simulink model "Motor_Postion_Ctrl"  (R2020a)
settings: Solver=VariableStepAuto  StartTime=0.0  StopTime=10.0  RelTol=1e-3
undefined symbols (not defined in the file): b, J, K, L, R
settings Model: DataDictionary=Motor_data.sldd  Creator=NIKITA  LastModifiedBy=NIKITA

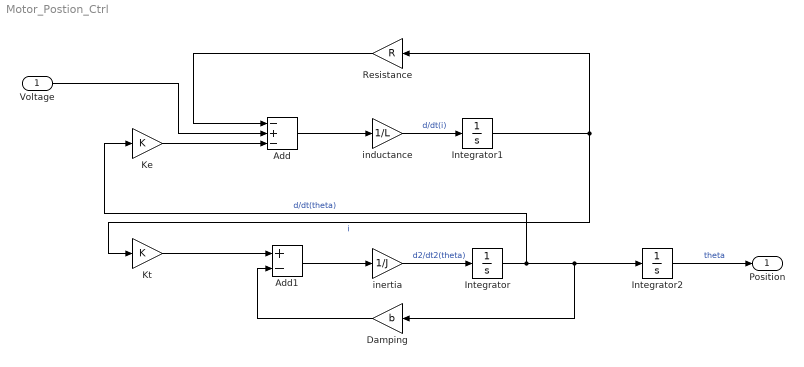
== system Motor_Postion_Ctrl ==
  Voltage : Inport
  Add : Sum  Inputs=-+-
  Add1 : Sum  Inputs=+-
  Damping : Gain  Gain=b
  "Integrator " : Integrator
  "Integrator1 " : Integrator
  Integrator2 : Integrator
  Ke : Gain  Gain=K
  Kt : Gain  Gain=K
  Resistance : Gain  Gain=R
  inductance : Gain  Gain=1/L
  inertia : Gain  Gain=1/J
  Position : Outport
  wires:
  inductance/1 -> "Integrator1 "/1  "d/dt(i)"
  "Integrator1 "/1 -> Resistance/1, Kt/1  "i"
  Integrator2/1 -> Position/1  "theta"
  Resistance/1 -> Add/1
  Kt/1 -> Add1/1
  Voltage/1 -> Add/2
  Add1/1 -> inertia/1
  inertia/1 -> "Integrator "/1  "d2/dt2(theta)"
  Damping/1 -> Add1/2
  "Integrator "/1 -> Ke/1, Integrator2/1, Damping/1  "d/dt(theta)"
  Ke/1 -> Add/3
  Add/1 -> inductance/1
